simulink model "ExampleQPKWIK"  (Simulink 8.2)
settings: Solver=ode15s  StartTime=0.0  StopTime=1  MaxStep=0.01  RelTol=1e-3
settings Model: Creator=Matze  LastModifiedBy=Re
settings DataIOCC: LimitDataPoints=off  SaveOutput=off  SignalLogging=off  DSMLogging=off  SaveTime=off
settings DebuggingCC: InheritedTsInSrcMsg=none
settings SFSimCC: SimParseCustomCode=off

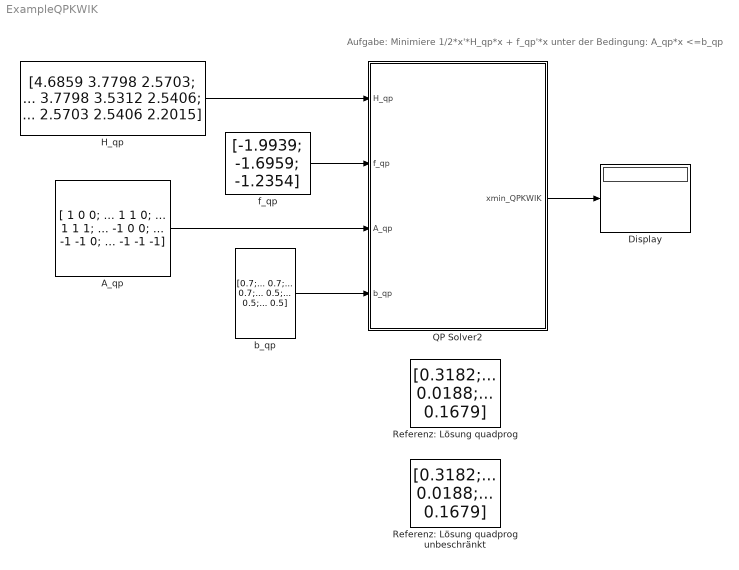
== system ExampleQPKWIK ==
  note: Aufgabe: Minimiere 1/2*x'*H_qp*x + f_qp'*x unter der Bedingung: A_qp*x <=b_qp
  A_qp : Constant  Value=|  VectorParams1D=off
      | [ 1     0     0; ...
      |          1     1     0; ...
      |          1     1     1; ...
      |         -1     0     0; ...
      |         -1    -1     0; ...
      |         -1    -1    -1]
  Display : Display
  H_qp : Constant  Value=|  VectorParams1D=off
      | [4.6859 3.7798 2.5703; ...
      |        3.7798 3.5312 2.5406; ...
      |        2.5703 2.5406 2.2015]
  QP Solver2 : MATLAB Function  TreatAsAtomicUnit=on
  Referenz: Lösung quadprog : Constant  Value=|  VectorParams1D=off
      | [0.3182;...
      |               0.0188;...
      |               0.1679]
  "Referenz: Lösung quadprog unbeschränkt " : Constant  Value=|  VectorParams1D=off
      | [0.3182;...
      |               0.0188;...
      |               0.1679]
  b_qp : Constant  Value=|  VectorParams1D=off
      | [0.7;...
      |        0.7;...
      |        0.7;... 
      |        0.5;... 
      |        0.5;...
      |        0.5]
  f_qp : Constant  Value=[-1.9939; -1.6959; -1.2354]  VectorParams1D=off
  wires:
  f_qp/1 -> QP Solver2/2(f_qp)
  H_qp/1 -> QP Solver2/1(H_qp)
  A_qp/1 -> QP Solver2/3(A_qp)
  b_qp/1 -> QP Solver2/4(b_qp)
  QP Solver2/1(xmin_QPKWIK) -> Display/1

== matlab function QP Solver2 ==
  settings: updateMethod=DISCRETE
  data: H_qp input double; f_qp input double; A_qp input double; b_qp input double; xmin_QPKWIK output double
function xmin_QPKWIK  = SolveQP(H_qp,f_qp, A_qp, b_qp)
Hu = size(H_qp,2);

%  ------------------------------------------------------------------------
%% Definition of Persistent variable iA (can be used to speed up in certain cases)
%  ------------------------------------------------------------------------
persistent iA 
if ( isempty(iA) )
    iA = false(length(A_qp)+Hu+1,1);
end

%  ------------------------------------------------------------------------
%% Setup Matrices for QP-Problem
%  ------------------------------------------------------------------------
Linv = chol(H_qp,'lower');
Linv = Linv\eye(Hu);
Hinv = Linv'*Linv;

maxiter = 120;
%xmin_QPKWIK = 0;

%  ------------------------------------------------------------------------
%% Solve QP-Problem
%  ------------------------------------------------------------------------
[xmin_QPKWIK,~,status,iA] = qpkwik_fixedsize(Linv,Hinv,f_qp,-A_qp,-b_qp,iA,maxiter); 
%%%%%%%%%%%%%%%%%%%%%%%%%%%%%%%%%%%%%%%%%%%%%%%%%%%%%%%%%%%%%%%%%%%%%%%%%
